simulink model "ncd_estim_1"  (Simulink 4.00)
settings: Solver=ode45  StartTime=0.0  StopTime=50.0  RelTol=1e-3
values from neighbouring files (symbols this model uses):
  A = my_sys1.a    [ncd_estim1.m]    (also in ncd_estim_1.mat = [-0.48 2 0 0 0 0 -1.0376 0 1 0 0 0 ... (36 elements, 6x6)]; ncd_kalm1.m; ncd_kalm2.m; ncd_kalm_1.mat = [-0.48 2 0 0 0 0 -1.0376 0 1 0 0 0 ... (36 elements, 6x6)])
  B = my_sys1.b    [ncd_estim1.m]    (also in ncd_estim_1.mat = [0.5 0 0 0 0 0]; ncd_kalm1.m; ncd_kalm2.m; ncd_kalm_1.mat = [0.5 0 0 0 0 0])
  C = my_sys1.c    [ncd_estim1.m]    (also in ncd_estim_1.mat = [0 0 0 0 0 0.4608]; ncd_kalm1.m; ncd_kalm2.m; ncd_kalm_1.mat = [0 0 0 0 0 0.4608])
  D = my_sys1.d    [ncd_estim1.m]    (also in ncd_estim_1.mat = 0; ncd_kalm1.m; ncd_kalm2.m; ncd_kalm_1.mat = 0)
  ki = 1    [ncd_estim1.m]    (also in ncd_estim_1.mat = 1.82974576844; ncd_kalm1.m; ncd_kalm2.m; ncd_kalm_1.mat = 1.97821802246)
  L = place(A, B, p)'    [ncd_estim1.m]    (also in ncd_estim_1.mat = [29.04 93.6748 304.13176 464.47352 317.56952 149.5392]; ncd_kalm_2.mat = [29.04 93.6748 304.13176 464.47352 317.56952 149.5392]; torce11.m = axis; torcell.mat = [0 100 0 3])
settings Model: LastModifiedBy=Administrator  BlockReductionOpt=off

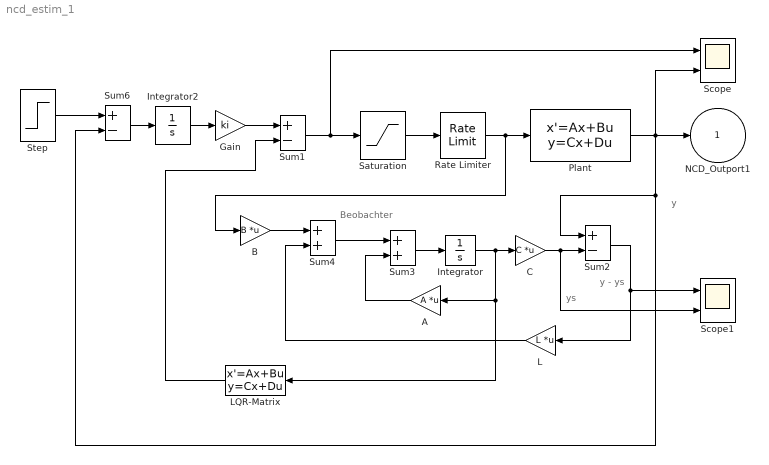
== system ncd_estim_1 ==
  note: Beobachter
  note: y
  note: ys
  note: y - ys
  A : Gain  Orientation=left  Gain=A  Multiplication=Matrix(K*u)  SaturateOnIntegerOverflow=on
  B : Gain  Gain=B  Multiplication=Matrix(K*u)  SaturateOnIntegerOverflow=on
  C : Gain  Gain=C  Multiplication=Matrix(K*u)  SaturateOnIntegerOverflow=on
  Gain : Gain  Gain=ki  Multiplication=Element-wise(K.*u)  SaturateOnIntegerOverflow=on
  Integrator : Integrator  ExternalReset=none  InitialConditionSource=internal  InitialCondition=0  LimitOutput=off  UpperSaturationLimit=inf  LowerSaturationLimit=-inf  ShowSaturationPort=off  ShowStatePort=off  AbsoluteTolerance=auto
  Integrator2 : Integrator  ExternalReset=none  InitialConditionSource=internal  InitialCondition=0  LimitOutput=off  UpperSaturationLimit=inf  LowerSaturationLimit=-inf  ShowSaturationPort=off  ShowStatePort=off  AbsoluteTolerance=auto
  L : Gain  Orientation=left  Gain=L  Multiplication=Matrix(K*u)  SaturateOnIntegerOverflow=on
  LQR-Matrix : StateSpace  Orientation=left  A=[]  B=[]  C=[]  D=K  X0=0  Realization=auto  AbsoluteTolerance=auto  mask(Matrix gain){@1=[k1, k2, k3, k4, k5, k6]}
      mask prompts: @1 "Gain matrix:"
      mask help: Matrix Gain:
      mask init:
      | K = @1;
      mask Help: Multiplies input vector by entered matrix to produce output vector.
      mask Display: disp('K')
  Plant : StateSpace  A=A  B=B  C=C  D=D  X0=0  Realization=auto  AbsoluteTolerance=auto
  Rate Limiter : RateLimiter  RisingSlewLimit=10  FallingSlewLimit=-10
  Saturation : Saturate  UpperLimit=1  LowerLimit=-1  LinearizeAsGain=on
  Scope : Scope  NumInputPorts=2
      settings: TimeRange=auto  YMin=-5~-5  YMax=5~5  SaveToWorkspace=off  SaveName=ScopeData  MaxDataPoints=5000
  Scope1 : Scope  NumInputPorts=2
      settings: TimeRange=auto  YMin=-5~-5  YMax=5~5  SaveToWorkspace=off  MaxDataPoints=5000
  Step : Step  Time=0  Before=0  After=1  SampleTime=0
  Sum1 : Sum  Inputs=+-  SaturateOnIntegerOverflow=on
  Sum2 : Sum  Inputs=+-  SaturateOnIntegerOverflow=on
  Sum3 : Sum  Inputs=++  SaturateOnIntegerOverflow=on
  Sum4 : Sum  Inputs=++  SaturateOnIntegerOverflow=on
  Sum6 : Sum  Inputs=+-  SaturateOnIntegerOverflow=on
  NCD_Outport1 : Outport  Port=1  InitialOutput=0
      settings: OpenFcn=optblock
      mask Type: NCD Outport
      mask Display:
      | plot([0:10],[-.5 1.5 .6 1.3 .8 1.1 .95 1.02 .99 1 1]);
      | disp('\n\n NCD\n OutPort 1');
  wires:
  Gain/1 -> Sum1/1
  LQR-Matrix/1 -> Sum1/2
  Rate Limiter/1 -> Plant/1, B/1
  Saturation/1 -> Rate Limiter/1
  Sum1/1 -> Saturation/1, Scope/1
  Step/1 -> Sum6/1
  Sum6/1 -> Integrator2/1
  Integrator2/1 -> Gain/1
  Plant/1 -> NCD_Outport1/1, Scope/2, Sum6/2, Sum2/1
  C/1 -> Sum2/2, Scope1/2
  Sum3/1 -> Integrator/1
  Integrator/1 -> C/1, A/1, LQR-Matrix/1
  A/1 -> Sum3/2
  Sum2/1 -> L/1, Scope1/1
  B/1 -> Sum4/1
  Sum4/1 -> Sum3/1
  L/1 -> Sum4/2
